simulink model "Test3"  (R2018b)
settings: Solver=VariableStepAuto  StartTime=0.0  StopTime=5e-6  RelTol=1e-3
model workspace (MAT data in the model file):
  a_1 = 0
  a_2 = 0
  delta = 0.001
values from neighbouring files (symbols this model uses):
  A = 1e-6    (= 1e-06)    [IC_4DOF_new.m]    (also in IC_4DOF_new2.m; ODE_4DOF_new.m = [zeros(4), eye(4); C+Hs, omega_dim*G+Hd/omega_dim]; ODE_MAGLEV_4DOF.m = [zeros(4), eye(4); C+Hs, (omega_dim*G)+(Hd/omega_dim)]; PID_Test2_.m = [zeros(4), eye(4); C+Hs, (omega_dim*G)+(Hd/omega_dim)])
  a1_dim = a1/Sl    (= 0.409090909091)    [IC_4DOF_new.m]    (also in IC_4DOF_new2.m; PID_Test2_.m; var_IC_4DOF.m)
  a2_dim = a2/Sl    (= 0.409090909091)    [IC_4DOF_new.m]    (also in IC_4DOF_new2.m; PID_Test2_.m; var_IC_4DOF.m)
  Ax_dim = Ax/Sf    (= 0.000833333333333)    [IC_4DOF_new.m]    (also in IC_4DOF_new2.m; PID_Test2_.m; var_IC_4DOF.m)
  delta_dim = delta_dim/Sx    (= 1)    [IC_4DOF_new.m]    (also in IC_4DOF_new2.m; PID_Test2_.m; var_IC_4DOF.m)
  h = 0.2*1e-3    (= 0.0002)    [IC_4DOF_new.m]    (also in IC_4DOF_new2.m; PID_Test2_.m; var_IC_4DOF.m)
  h_dim = h/Sl    (= 0.00909090909091)    [IC_4DOF_new.m]    (also in IC_4DOF_new2.m; PID_Test2_.m; var_IC_4DOF.m)
  i0_dim = i0/Si    (= 0)    [IC_4DOF_new.m]    (also in IC_4DOF_new2.m = 0.05; PID_Test2_.m = 0.0007; var_IC_4DOF.m = 0.5)
  omega_dim = omega/Sw    [IC_4DOF_new.m]    (also in IC_4DOF_new2.m; ODE_4DOF_new.m = par(11); ODE_MAGLEV_4DOF.m = par(11); PID_Test2_.m)
  P2 = par(22)    [Force_4DOF.m]    (also in IC_4DOF_new.m = 2.178; IC_4DOF_new2.m = 2.178; PID_Test2_.m = 8.714; var_IC_4DOF.m = 2.178)
  p_dim = nu*2*pi/Sw    [AFC_4DOF_NM.m]    (also in IC_4DOF_new.m = p/Sw; IC_4DOF_new2.m = p/Sw; PID_Test2_.m = p/Sw; var_IC_4DOF.m = p/Sw)
  Pk = par(15)    [Force_4DOF.m]    (also in IC_4DOF_new.m = 8.41666666667e-05; IC_4DOF_new2.m = ka*P_e/(cm*R_e*delta_dim^3); PID_Test2_.m = 1000000; var_IC_4DOF.m = ka*P_e/(cm*R_e*delta_dim^3))
  Px_dim = Px/Sf    (= 0)    [IC_4DOF_new.m]    (also in IC_4DOF_new2.m = 1.62337662338; PID_Test2_.m; var_IC_4DOF.m)
  Zb = [1 0 0 -a1_dim ... (first row only)    [IC_4DOF_new.m]    (also in IC_4DOF_new2.m; PID_Test2_.m; var_IC_4DOF.m)
libraries: simulink x25, cstblocks x1, neural x1
settings Model: Creator=Vladimir  LastModifiedBy=first
settings SolverCC: AlgebraicLoopSolver=LineSearch

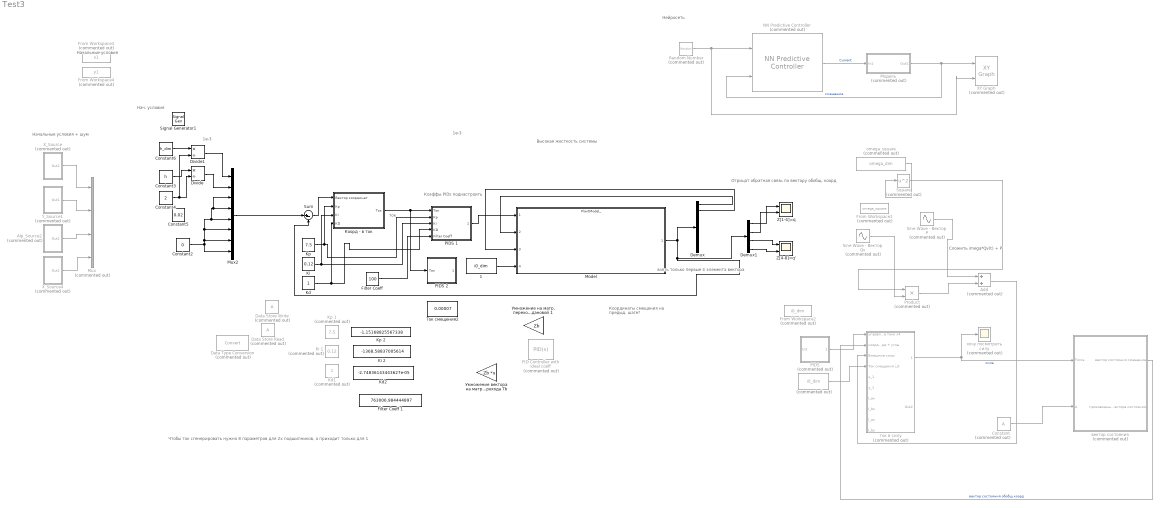
== system Test3 ==
  note: 1e-3
  note: Нач. условия
  note: 1e-3
  note: Высокая жесткость системы
  note: Коэффы PIDs поднастроить
  note: Чтобы ток сгенерировать нужно 8 параметров для 2х подшипников, а приходит только для 1
  note: Координаты смещения
      | на предыд. шаге?
  note: взять только первые 4 элемента вектора
  note: Нейросеть
  note: Начальные условия
  note: Отрицат обратная связь по вектору обобщ. коорд
  note: Сложить imega*Qv(t) + P
  note: Начальные условия + шум
  note: ток
  " " : Constant  Commented=on  Value=i0_dim
  " 1" : Constant  Value=i0_dim
  " Ток смещения2" : Constant  Value=0.00007
  " вектор состояния " : Subsystem  Commented=on
  Add : Sum  Commented=on
  Alp_Source2 : Subsystem  Commented=on
  Constant : Constant  Commented=on  Value=A
  Constant2 : Constant  Value=0
  Constant3 : Constant  Value=h
  Constant4 : Constant  Value=2
  Constant5 : Constant  Value=0.02
  Constant6 : Constant  Value=h_dim
  Data Store Read : DataStoreRead  Commented=on
  Data Store Write : DataStoreWrite  Commented=on
  Data Type Conversion : DataTypeConversion  Commented=on
  Demux : Demux  Outputs=8
  Demux1 : Demux
  Divide : Product  Inputs=*/
  Divide1 : Product  Inputs=*/
  "Filter Coeff " : Constant  Value=100
  Filter Coeff 1 : Constant  Value=763006.984444897
  From Workspace1 : FromWorkspace  Commented=on  VariableName=omega_square  SampleTime=0
  From Workspace2 : FromWorkspace  Commented=on  VariableName=i0_dim  SampleTime=0
  From Workspace3 : FromWorkspace  Commented=on  VariableName=x1  SampleTime=0
  From Workspace4 : FromWorkspace  Commented=on  VariableName=y1  SampleTime=0
  Kd : Constant
  Kd1 : Constant  Commented=on
  Kd2 : Constant  Value=-2.74836143443627e-05
  "Ki " : Constant  Value=0.12
  Ki 1 : Constant  Commented=on  Value=0.12
  Ki 2 : Constant  Value=-1368.58837005614
  "Kp " : Constant  Value=7.5
  Kp 1 : Constant  Commented=on  Value=7.5
  Kp 2 : Constant  Value=-1.15168825567338
  Model : ModelReference  ModelNameDialog=PlantModel_.slx  SimulationMode=Normal  ModelReferenceVersion=1.31
  Mux : Mux  Commented=on
  Mux2 : Mux  Inputs=8
  NN Predictive Controller : neural/Control Systems/NN Predictive Controller  Commented=on  epochs=500  minp=[]  maxp=[]  mint=[]  maxt=[]  Normalize=[]  IW=[]  LW1_2=[]  LW2_1=[]  B1=[]  B2=[]  max_i_int=[]  min_i_int=[]  limit_output=[]  max_output=[]  min_output=[]  Use_Previous_Weights=[]  N2=7  Nu=2  Ts=[]  rho=0.05  alpha=0.001  csrchfun=csrchbac  maxiter=2  S1=[]  Ni=[]  Nj=[]  sim_file=0  trainfun=trainlm  Use_validation=[]  Use_Testing=[]  max_i=[]  min_i=[]  sam_training=[]
      settings: SourceProductName=Neural Network Toolbox  SourceProductBaseCode=NN
  "PID Controller with ideal coeff " : simulink/Continuous/PID Controller  Commented=on  Controller=PID  Form=Parallel  TimeDomain=Continuous-time  SampleTime=-1  IntegratorMethod=Forward Euler  FilterMethod=Forward Euler  ControllerParametersSource=internal  P=7.5  I=0.12  D=1  UseFilter=on  N=100  TunerSelectOption=Transfer Function Based (PID Tuner App)  InitialConditionSource=internal  InitialConditionForIntegrator=0  InitialConditionForFilter=0  DifferentiatorICPrevScaledInput=0  ExternalReset=none  TrackingMode=off  Kt=1  LimitOutput=off  UpperSaturationLimit=inf  LowerSaturationLimit=-inf  LinearizeAsGain=on  AntiWindupMode=none  Kb=1  POutMin=[]  POutMax=[]  IOutMin=[]  IOutMax=[]  DOutMin=[]  DOutMax=[]  NOutMin=[]  NOutMax=[]  SumOutMin=[]  SumOutMax=[]  SaturationOutMin=[]  SaturationOutMax=[]  PParamMin=[]  PParamMax=[]  IParamMin=[]  IParamMax=[]  DParamMin=[]  DParamMax=[]  NParamMin=[]  NParamMax=[]  KbParamMin=[]  KbParamMax=[]  KtParamMin=[]  KtParamMax=[]  KbOutMin=[]  KbOutMax=[]  KtOutMin=[]  KtOutMax=[]  IntegratorOutMin=[]  IntegratorOutMax=[]  FilterOutMin=[]  FilterOutMax=[]  SumI1OutMin=[]  SumI1OutMax=[]  SumI2OutMin=[]  SumI2OutMax=[]  SumI3OutMin=[]  SumI3OutMax=[]  SumI4OutMin=[]  SumI4OutMax=[]  SumDOutMin=[]  SumDOutMax=[]  DifferentiatorOutMin=[]  DifferentiatorOutMax=[]  FilterDiffOutCoefMin=[]  FilterDiffOutCoefMax=[]  ReciprocalOutMin=[]  ReciprocalOutMax=[]  SumDenOutMin=[]  SumDenOutMax=[]  SumNumOutMin=[]  SumNumOutMax=[]  DivideOutMin=[]  DivideOutMax=[]  IntegratorContinuousStateAttributes=''  IntegratorStateMustResolveToSignalObject=off  IntegratorRTWStateStorageClass=Auto  FilterContinuousStateAttributes=''  FilterStateMustResolveToSignalObject=off  FilterRTWStateStorageClass=Auto  ParallelPVariant=InternalParameters  IdealPVariant=Disabled  IVariant=InternalParameters  DVariant=InternalParameters  IntegratorVariant=Continuous  SatVariant=Disabled  AWVariant=Passthrough  PCopyVariant=Disabled  TRVariant=Disabled  FdbkBlocksVariant=Forward  IdealPFdbkVariant=Disabled  SatFdbkVariant=Disabled  DerivativeFilterVariant=ContFilter  NVariant=InternalParameters  NCopyVariant=Disabled  FilterICVariant=InternalICsFilter  IntegratorICVariant=InternalICs  ExternalResetVariant=Disabled  TRSumVariant=Passthrough  SumFdbkVariant=Disabled  SumVariant=Sum_PID
  "PIDS " : Subsystem  Commented=on
  PIDS 1 : Subsystem
  PIDS 2 : Subsystem
  Product : Product  Commented=on
  Random Number : RandomNumber  Commented=on  SampleTime=0.1
  Signal Generator1 : SignalGenerator  Amplitude=h/2  Units=rad/sec
  Sine Wave - Вектор P : Sin  Commented=on  Amplitude=Ax_dim  Bias=Px_dim  Frequency=p_dim  SampleTime=1
  Sine Wave - Вектор Qv : Sin  Commented=on  Amplitude=Ax_dim  Bias=Px_dim  Frequency=p_dim  SampleTime=1
  Square : Math  Commented=on  Operator=square  SaturateOnIntegerOverflow=on
  Sum : Sum  Inputs=|+-
  XY Graph : simulink/Sinks/XY Graph  Commented=on  xmin=-1  xmax=1  ymin=-1  ymax=1  st=-1
  X_Source : Subsystem  Commented=on
  X_Source4 : Subsystem  Commented=on
  Y_Source1 : Subsystem  Commented=on
  "Z[1-4]=q " : Scope  NumInputPorts=2
  Z[4-8]=q' : Scope  NumInputPorts=2
  omega_square : Constant  Commented=on  Value=omega_dim
  "Коорд - в ток " : Subsystem
  "Модель " : Subsystem  Commented=on
  "Умножение вектора на матр. перехода Tb " : Gain  Gain=Zb  Multiplication=Matrix(K*u) (u vector)
  "Умножение на матр. перехода Tb, посмотреть у Богдановой 1" : Gain  Gain=Zb
  "ток в силу " : Subsystem  Commented=on
  хочу посмотреть силу : Scope  Commented=on
  wires:
  X_Source/1(Out1) -> Mux/1
  Y_Source1/1(Out1) -> Mux/2
  Alp_Source2/1(Out1) -> Mux/3
  X_Source4/1(Out1) -> Mux/4
  " вектор состояния "/1(вектор состояния смещение) -> "ток в силу "/2(координаты на предидущий такт коорд + углы)  "вектор состояния обобщ коорд"
  "ток в силу "/1(" ") -> хочу посмотреть силу/1, " вектор состояния "/1(Force)  "сила"
  Demux1/1 -> "Z[1-4]=q "/1
  Demux1/2 -> "Z[1-4]=q "/2
  Demux1/3 -> Z[4-8]=q'/1
  Demux1/4 -> Z[4-8]=q'/2
  Add/1 -> "ток в силу "/3(Внешние силы)
  Sine Wave - Вектор P/1 -> Add/1
  "PIDS "/1("  ") -> "ток в силу "/1(управляющие токи x4)
  Sine Wave - Вектор Qv/1 -> Product/2
  Product/1 -> Add/2
  " "/1 -> "ток в силу "/4(Ток смещения i_0)
  Constant/1 -> " вектор состояния "/2("A ")
  omega_square/1 -> Square/1
  Square/1 -> Product/1
  Sum/1 -> "Коорд - в ток "/1(Вектор координат)
  Random Number/1 -> XY Graph/2, NN Predictive Controller/1
  NN Predictive Controller/1 -> "Модель "/1(In1)  "Current"
  "Модель "/1(Out1) -> NN Predictive Controller/2, XY Graph/1  "смещение"
  Model/1 -> Demux1/1, Sum/2, Demux/1
  "Коорд - в ток "/1(Ток) -> PIDS 2/1(Ток), PIDS 1/1(Ток)
  Demux/1 -> Model/2
  Demux/2 -> Model/3
  Constant2/1 -> Mux2/8, Mux2/6, Mux2/3, Mux2/4, Mux2/5, Mux2/7
  Mux2/1 -> Sum/1
  Constant4/1 -> Divide1/2, Divide/2
  "Kp "/1 -> "Коорд - в ток "/2(Kp), PIDS 1/2(Kp)
  "Ki "/1 -> PIDS 1/3(Ki), "Коорд - в ток "/3(Ki)
  Kd/1 -> PIDS 1/4("KD "), "Коорд - в ток "/4("KD ")
  "Filter Coeff "/1 -> PIDS 1/5(Filter Coeff)
  " 1"/1 -> Model/4
  PIDS 1/1("  ") -> Model/1
  Constant3/1 -> Divide/1
  Constant6/1 -> Divide1/1
  Divide1/1 -> Mux2/1
  Divide/1 -> Mux2/2

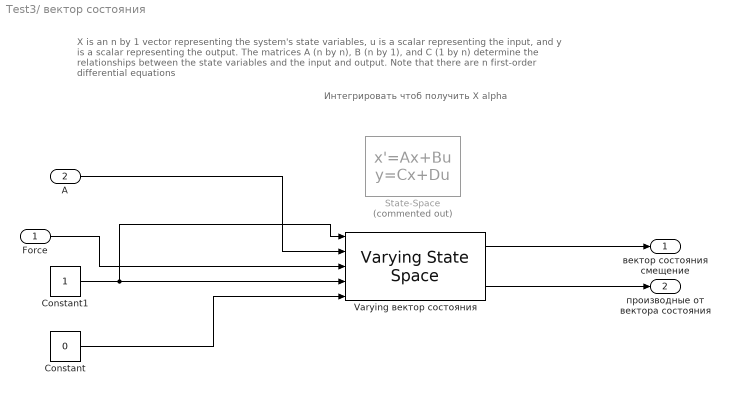
== system Test3/ вектор состояния  ==
  note: X is an n by 1 vector representing the system's state variables, u is a scalar representing the input, and y is a scalar representing the output.
      |  The matrices A (n by n), B (n by 1), and C (1 by n) determine the relationships between the state variables and the input and output.
      | Note that there are n first-order differential equations
  note: Интегрировать чтоб получить X alpha
  Force : Inport
  "A " : Inport  Port=2
  Constant : Constant  Value=0
  Constant1 : Constant
  State-Space : StateSpace  Commented=on  InitialCondition=0
  Varying вектор состояния : cstblocks/Linear Parameter Varying/Varying State Space  x0=0  xNames=''  OutputX=on  OutputDX=on
      settings: SourceProductName=Control System Toolbox
  вектор состояния смещение : Outport
  производные от вектора состояния : Outport  Port=2
  wires:
  Force/1 -> Varying вектор состояния/3
  "A "/1 -> Varying вектор состояния/2
  Varying вектор состояния/3 -> производные от вектора состояния/1
  Constant/1 -> Varying вектор состояния/5
  Constant1/1 -> Varying вектор состояния/4, Varying вектор состояния/1
  Varying вектор состояния/1 -> вектор состояния смещение/1

== system Test3/Alp_Source2 ==
  note: Tok Here
  note: dtrnjh 4[
  Band-Limited White Noise : simulink/Sources/Band-Limited White Noise  Cov=[0.1]  Ts=0.1  seed=[23341]
  Gain : Gain
  Gain1 : Gain
  Sine Wave : Sin  SampleTime=0
  Step : Step  SampleTime=0
  Sum : Sum  Inputs=|+++
  Out1 : Outport
  wires:
  Gain1/1 -> Sum/3
  Band-Limited White Noise/1 -> Gain/1
  Sine Wave/1 -> Gain1/1
  Step/1 -> Sum/1
  Gain/1 -> Sum/2
  Sum/1 -> Out1/1

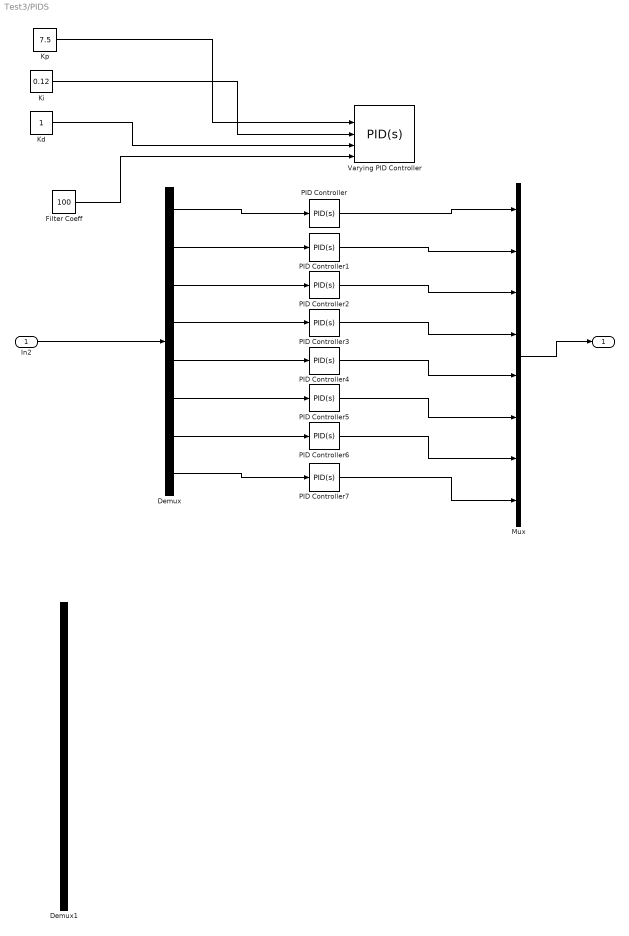
== system Test3/PIDS  ==
  In2 : Inport
  Demux : Demux  Outputs=8
  Demux1 : Demux  Outputs=8
  "Filter Coeff " : Constant  Value=100
  Kd : Constant
  "Ki " : Constant  Value=0.12
  "Kp " : Constant  Value=7.5
  Mux : Mux  Inputs=8
  PID Controller{,1..7} (8 alike) : simulink/Continuous/PID Controller  Controller=PID  Form=Parallel  TimeDomain=Continuous-time  SampleTime=-1  IntegratorMethod=Forward Euler  FilterMethod=Forward Euler  ControllerParametersSource=internal  P=1  I=1  D=0  UseFilter=on  N=100  TunerSelectOption=Transfer Function Based (PID Tuner App)  InitialConditionSource=internal  InitialConditionForIntegrator=0  InitialConditionForFilter=0  DifferentiatorICPrevScaledInput=0  ExternalReset=none  TrackingMode=off  Kt=1  LimitOutput=off  UpperSaturationLimit=inf  LowerSaturationLimit=-inf  LinearizeAsGain=on  AntiWindupMode=none  Kb=1  POutMin=[]  POutMax=[]  IOutMin=[]  IOutMax=[]  DOutMin=[]  DOutMax=[]  NOutMin=[]  NOutMax=[]  SumOutMin=[]  SumOutMax=[]  SaturationOutMin=[]  SaturationOutMax=[]  PParamMin=[]  PParamMax=[]  IParamMin=[]  IParamMax=[]  DParamMin=[]  DParamMax=[]  NParamMin=[]  NParamMax=[]  KbParamMin=[]  KbParamMax=[]  KtParamMin=[]  KtParamMax=[]  KbOutMin=[]  KbOutMax=[]  KtOutMin=[]  KtOutMax=[]  IntegratorOutMin=[]  IntegratorOutMax=[]  FilterOutMin=[]  FilterOutMax=[]  SumI1OutMin=[]  SumI1OutMax=[]  SumI2OutMin=[]  SumI2OutMax=[]  SumI3OutMin=[]  SumI3OutMax=[]  SumI4OutMin=[]  SumI4OutMax=[]  SumDOutMin=[]  SumDOutMax=[]  DifferentiatorOutMin=[]  DifferentiatorOutMax=[]  FilterDiffOutCoefMin=[]  FilterDiffOutCoefMax=[]  ReciprocalOutMin=[]  ReciprocalOutMax=[]  SumDenOutMin=[]  SumDenOutMax=[]  SumNumOutMin=[]  SumNumOutMax=[]  DivideOutMin=[]  DivideOutMax=[]  IntegratorContinuousStateAttributes=''  IntegratorStateMustResolveToSignalObject=off  IntegratorRTWStateStorageClass=Auto  FilterContinuousStateAttributes=''  FilterStateMustResolveToSignalObject=off  FilterRTWStateStorageClass=Auto  ParallelPVariant=InternalParameters  IdealPVariant=Disabled  IVariant=InternalParameters  DVariant=InternalParameters  IntegratorVariant=Continuous  SatVariant=Disabled  AWVariant=Passthrough  PCopyVariant=Disabled  TRVariant=Disabled  FdbkBlocksVariant=Forward  IdealPFdbkVariant=Disabled  SatFdbkVariant=Disabled  DerivativeFilterVariant=ContFilter  NVariant=InternalParameters  NCopyVariant=Disabled  FilterICVariant=InternalICsFilter  IntegratorICVariant=InternalICs  ExternalResetVariant=Disabled  TRSumVariant=Passthrough  SumFdbkVariant=Disabled  SumVariant=Sum_PID
  Varying PID Controller : simulink/Continuous/PID Controller  Controller=PID  Form=Parallel  TimeDomain=Continuous-time  SampleTime=-1  IntegratorMethod=Forward Euler  FilterMethod=Forward Euler  ControllerParametersSource=external  P=1  I=1  D=0  UseFilter=on  N=100  TunerSelectOption=Transfer Function Based (PID Tuner App)  InitialConditionSource=internal  InitialConditionForIntegrator=0  InitialConditionForFilter=0  DifferentiatorICPrevScaledInput=0  ExternalReset=none  TrackingMode=off  Kt=1  LimitOutput=off  UpperSaturationLimit=inf  LowerSaturationLimit=-inf  LinearizeAsGain=on  AntiWindupMode=none  Kb=1  POutMin=[]  POutMax=[]  IOutMin=[]  IOutMax=[]  DOutMin=[]  DOutMax=[]  NOutMin=[]  NOutMax=[]  SumOutMin=[]  SumOutMax=[]  SaturationOutMin=[]  SaturationOutMax=[]  PParamMin=[]  PParamMax=[]  IParamMin=[]  IParamMax=[]  DParamMin=[]  DParamMax=[]  NParamMin=[]  NParamMax=[]  KbParamMin=[]  KbParamMax=[]  KtParamMin=[]  KtParamMax=[]  KbOutMin=[]  KbOutMax=[]  KtOutMin=[]  KtOutMax=[]  IntegratorOutMin=[]  IntegratorOutMax=[]  FilterOutMin=[]  FilterOutMax=[]  SumI1OutMin=[]  SumI1OutMax=[]  SumI2OutMin=[]  SumI2OutMax=[]  SumI3OutMin=[]  SumI3OutMax=[]  SumI4OutMin=[]  SumI4OutMax=[]  SumDOutMin=[]  SumDOutMax=[]  DifferentiatorOutMin=[]  DifferentiatorOutMax=[]  FilterDiffOutCoefMin=[]  FilterDiffOutCoefMax=[]  ReciprocalOutMin=[]  ReciprocalOutMax=[]  SumDenOutMin=[]  SumDenOutMax=[]  SumNumOutMin=[]  SumNumOutMax=[]  DivideOutMin=[]  DivideOutMax=[]  IntegratorContinuousStateAttributes=''  IntegratorStateMustResolveToSignalObject=off  IntegratorRTWStateStorageClass=Auto  FilterContinuousStateAttributes=''  FilterStateMustResolveToSignalObject=off  FilterRTWStateStorageClass=Auto  ParallelPVariant=ExternalParameters  IdealPVariant=Disabled  IVariant=ExternalParameters  DVariant=ExternalParameters  IntegratorVariant=Continuous  SatVariant=Disabled  AWVariant=Passthrough  PCopyVariant=Disabled  TRVariant=Disabled  FdbkBlocksVariant=Forward  IdealPFdbkVariant=Disabled  SatFdbkVariant=Disabled  DerivativeFilterVariant=ContFilter  NVariant=ExternalParameters  NCopyVariant=Disabled  FilterICVariant=InternalICsFilter  IntegratorICVariant=InternalICs  ExternalResetVariant=Disabled  TRSumVariant=Passthrough  SumFdbkVariant=Disabled  SumVariant=Sum_PID
  "  " : Outport
  wires:
  Demux/1 -> PID Controller/1
  Demux/2 -> PID Controller1/1
  Demux/3 -> PID Controller2/1
  Demux/4 -> PID Controller3/1
  In2/1 -> Demux/1
  Demux/5 -> PID Controller4/1
  Demux/6 -> PID Controller5/1
  Demux/7 -> PID Controller6/1
  Demux/8 -> PID Controller7/1
  PID Controller/1 -> Mux/1
  PID Controller1/1 -> Mux/2
  PID Controller2/1 -> Mux/3
  PID Controller3/1 -> Mux/4
  PID Controller4/1 -> Mux/5
  PID Controller5/1 -> Mux/6
  PID Controller6/1 -> Mux/7
  PID Controller7/1 -> Mux/8
  Mux/1 -> "  "/1
  "Kp "/1 -> Varying PID Controller/2
  "Filter Coeff "/1 -> Varying PID Controller/5
  "Ki "/1 -> Varying PID Controller/3
  Kd/1 -> Varying PID Controller/4

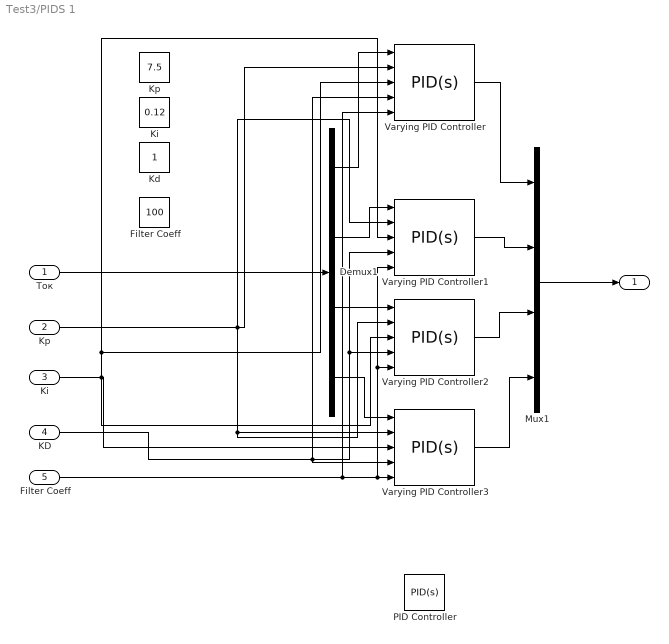
== system Test3/PIDS 1 ==
  Ток : Inport
  Kp : Inport  Port=2
  Ki : Inport  Port=3
  "KD " : Inport  Port=4
  Filter Coeff : Inport  Port=5
  Demux1 : Demux
  "Filter Coeff " : Constant  Value=100
  Kd : Constant
  "Ki " : Constant  Value=0.12
  "Kp " : Constant  Value=7.5
  Mux1 : Mux
  PID Controller : simulink/Continuous/PID Controller  Controller=PID  Form=Parallel  TimeDomain=Continuous-time  SampleTime=-1  IntegratorMethod=Forward Euler  FilterMethod=Forward Euler  ControllerParametersSource=internal  P=1  I=1  D=0  UseFilter=on  N=100  TunerSelectOption=Transfer Function Based (PID Tuner App)  InitialConditionSource=internal  InitialConditionForIntegrator=0  InitialConditionForFilter=0  DifferentiatorICPrevScaledInput=0  ExternalReset=none  TrackingMode=off  Kt=1  LimitOutput=off  UpperSaturationLimit=inf  LowerSaturationLimit=-inf  LinearizeAsGain=on  AntiWindupMode=none  Kb=1  POutMin=[]  POutMax=[]  IOutMin=[]  IOutMax=[]  DOutMin=[]  DOutMax=[]  NOutMin=[]  NOutMax=[]  SumOutMin=[]  SumOutMax=[]  SaturationOutMin=[]  SaturationOutMax=[]  PParamMin=[]  PParamMax=[]  IParamMin=[]  IParamMax=[]  DParamMin=[]  DParamMax=[]  NParamMin=[]  NParamMax=[]  KbParamMin=[]  KbParamMax=[]  KtParamMin=[]  KtParamMax=[]  KbOutMin=[]  KbOutMax=[]  KtOutMin=[]  KtOutMax=[]  IntegratorOutMin=[]  IntegratorOutMax=[]  FilterOutMin=[]  FilterOutMax=[]  SumI1OutMin=[]  SumI1OutMax=[]  SumI2OutMin=[]  SumI2OutMax=[]  SumI3OutMin=[]  SumI3OutMax=[]  SumI4OutMin=[]  SumI4OutMax=[]  SumDOutMin=[]  SumDOutMax=[]  DifferentiatorOutMin=[]  DifferentiatorOutMax=[]  FilterDiffOutCoefMin=[]  FilterDiffOutCoefMax=[]  ReciprocalOutMin=[]  ReciprocalOutMax=[]  SumDenOutMin=[]  SumDenOutMax=[]  SumNumOutMin=[]  SumNumOutMax=[]  DivideOutMin=[]  DivideOutMax=[]  IntegratorContinuousStateAttributes=''  IntegratorStateMustResolveToSignalObject=off  IntegratorRTWStateStorageClass=Auto  FilterContinuousStateAttributes=''  FilterStateMustResolveToSignalObject=off  FilterRTWStateStorageClass=Auto  ParallelPVariant=InternalParameters  IdealPVariant=Disabled  IVariant=InternalParameters  DVariant=InternalParameters  IntegratorVariant=Continuous  SatVariant=Disabled  AWVariant=Passthrough  PCopyVariant=Disabled  TRVariant=Disabled  FdbkBlocksVariant=Forward  IdealPFdbkVariant=Disabled  SatFdbkVariant=Disabled  DerivativeFilterVariant=ContFilter  NVariant=InternalParameters  NCopyVariant=Disabled  FilterICVariant=InternalICsFilter  IntegratorICVariant=InternalICs  ExternalResetVariant=Disabled  TRSumVariant=Passthrough  SumFdbkVariant=Disabled  SumVariant=Sum_PID
  Varying PID Controller{,1..3} (4 alike) : simulink/Continuous/PID Controller  Controller=PID  Form=Parallel  TimeDomain=Continuous-time  SampleTime=-1  IntegratorMethod=Forward Euler  FilterMethod=Forward Euler  ControllerParametersSource=external  P=1  I=1  D=0  UseFilter=on  N=100  TunerSelectOption=Transfer Function Based (PID Tuner App)  InitialConditionSource=internal  InitialConditionForIntegrator=0  InitialConditionForFilter=0  DifferentiatorICPrevScaledInput=0  ExternalReset=none  TrackingMode=off  Kt=1  LimitOutput=off  UpperSaturationLimit=inf  LowerSaturationLimit=-inf  LinearizeAsGain=on  AntiWindupMode=none  Kb=1  POutMin=[]  POutMax=[]  IOutMin=[]  IOutMax=[]  DOutMin=[]  DOutMax=[]  NOutMin=[]  NOutMax=[]  SumOutMin=[]  SumOutMax=[]  SaturationOutMin=[]  SaturationOutMax=[]  PParamMin=[]  PParamMax=[]  IParamMin=[]  IParamMax=[]  DParamMin=[]  DParamMax=[]  NParamMin=[]  NParamMax=[]  KbParamMin=[]  KbParamMax=[]  KtParamMin=[]  KtParamMax=[]  KbOutMin=[]  KbOutMax=[]  KtOutMin=[]  KtOutMax=[]  IntegratorOutMin=[]  IntegratorOutMax=[]  FilterOutMin=[]  FilterOutMax=[]  SumI1OutMin=[]  SumI1OutMax=[]  SumI2OutMin=[]  SumI2OutMax=[]  SumI3OutMin=[]  SumI3OutMax=[]  SumI4OutMin=[]  SumI4OutMax=[]  SumDOutMin=[]  SumDOutMax=[]  DifferentiatorOutMin=[]  DifferentiatorOutMax=[]  FilterDiffOutCoefMin=[]  FilterDiffOutCoefMax=[]  ReciprocalOutMin=[]  ReciprocalOutMax=[]  SumDenOutMin=[]  SumDenOutMax=[]  SumNumOutMin=[]  SumNumOutMax=[]  DivideOutMin=[]  DivideOutMax=[]  IntegratorContinuousStateAttributes=''  IntegratorStateMustResolveToSignalObject=off  IntegratorRTWStateStorageClass=Auto  FilterContinuousStateAttributes=''  FilterStateMustResolveToSignalObject=off  FilterRTWStateStorageClass=Auto  ParallelPVariant=ExternalParameters  IdealPVariant=Disabled  IVariant=ExternalParameters  DVariant=ExternalParameters  IntegratorVariant=Continuous  SatVariant=Disabled  AWVariant=Passthrough  PCopyVariant=Disabled  TRVariant=Disabled  FdbkBlocksVariant=Forward  IdealPFdbkVariant=Disabled  SatFdbkVariant=Disabled  DerivativeFilterVariant=ContFilter  NVariant=ExternalParameters  NCopyVariant=Disabled  FilterICVariant=InternalICsFilter  IntegratorICVariant=InternalICs  ExternalResetVariant=Disabled  TRSumVariant=Passthrough  SumFdbkVariant=Disabled  SumVariant=Sum_PID
  "  " : Outport
  wires:
  Mux1/1 -> "  "/1
  Ток/1 -> Demux1/1
  Demux1/1 -> Varying PID Controller/1
  Varying PID Controller/1 -> Mux1/1
  Demux1/2 -> Varying PID Controller1/1
  Varying PID Controller1/1 -> Mux1/2
  Demux1/3 -> Varying PID Controller2/1
  Varying PID Controller2/1 -> Mux1/3
  Demux1/4 -> Varying PID Controller3/1
  Varying PID Controller3/1 -> Mux1/4
  Filter Coeff/1 -> Varying PID Controller/5, Varying PID Controller1/5, Varying PID Controller2/5, Varying PID Controller3/5
  "KD "/1 -> Varying PID Controller/4, Varying PID Controller1/4, Varying PID Controller2/4, Varying PID Controller3/4
  Ki/1 -> Varying PID Controller/3, Varying PID Controller1/3, Varying PID Controller2/3, Varying PID Controller3/3
  Kp/1 -> Varying PID Controller3/2, Varying PID Controller2/2, Varying PID Controller1/2, Varying PID Controller/2

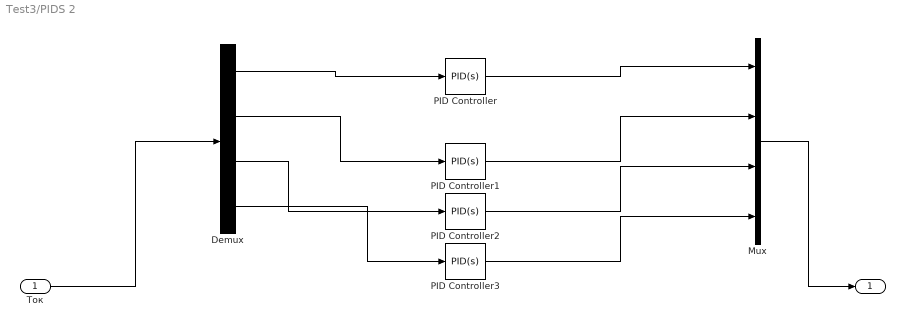
== system Test3/PIDS 2 ==
  Ток : Inport
  Demux : Demux
  Mux : Mux
  PID Controller : simulink/Continuous/PID Controller  Controller=PID  Form=Parallel  TimeDomain=Continuous-time  SampleTime=-1  IntegratorMethod=Forward Euler  FilterMethod=Forward Euler  ControllerParametersSource=internal  P=-1.15168825567338  I=-1368.58837005614  D=-2.74836143443627e-05  UseFilter=on  N=763006.984444897  TunerSelectOption=Transfer Function Based (PID Tuner App)  InitialConditionSource=internal  InitialConditionForIntegrator=0  InitialConditionForFilter=0  DifferentiatorICPrevScaledInput=0  ExternalReset=none  TrackingMode=off  Kt=1  LimitOutput=off  UpperSaturationLimit=inf  LowerSaturationLimit=-inf  LinearizeAsGain=on  AntiWindupMode=none  Kb=1  POutMin=[]  POutMax=[]  IOutMin=[]  IOutMax=[]  DOutMin=[]  DOutMax=[]  NOutMin=[]  NOutMax=[]  SumOutMin=[]  SumOutMax=[]  SaturationOutMin=[]  SaturationOutMax=[]  PParamMin=[]  PParamMax=[]  IParamMin=[]  IParamMax=[]  DParamMin=[]  DParamMax=[]  NParamMin=[]  NParamMax=[]  KbParamMin=[]  KbParamMax=[]  KtParamMin=[]  KtParamMax=[]  KbOutMin=[]  KbOutMax=[]  KtOutMin=[]  KtOutMax=[]  IntegratorOutMin=[]  IntegratorOutMax=[]  FilterOutMin=[]  FilterOutMax=[]  SumI1OutMin=[]  SumI1OutMax=[]  SumI2OutMin=[]  SumI2OutMax=[]  SumI3OutMin=[]  SumI3OutMax=[]  SumI4OutMin=[]  SumI4OutMax=[]  SumDOutMin=[]  SumDOutMax=[]  DifferentiatorOutMin=[]  DifferentiatorOutMax=[]  FilterDiffOutCoefMin=[]  FilterDiffOutCoefMax=[]  ReciprocalOutMin=[]  ReciprocalOutMax=[]  SumDenOutMin=[]  SumDenOutMax=[]  SumNumOutMin=[]  SumNumOutMax=[]  DivideOutMin=[]  DivideOutMax=[]  IntegratorContinuousStateAttributes=''  IntegratorStateMustResolveToSignalObject=off  IntegratorRTWStateStorageClass=Auto  FilterContinuousStateAttributes=''  FilterStateMustResolveToSignalObject=off  FilterRTWStateStorageClass=Auto  ParallelPVariant=InternalParameters  IdealPVariant=Disabled  IVariant=InternalParameters  DVariant=InternalParameters  IntegratorVariant=Continuous  SatVariant=Disabled  AWVariant=Passthrough  PCopyVariant=Disabled  TRVariant=Disabled  FdbkBlocksVariant=Forward  IdealPFdbkVariant=Disabled  SatFdbkVariant=Disabled  DerivativeFilterVariant=ContFilter  NVariant=InternalParameters  NCopyVariant=Disabled  FilterICVariant=InternalICsFilter  IntegratorICVariant=InternalICs  ExternalResetVariant=Disabled  TRSumVariant=Passthrough  SumFdbkVariant=Disabled  SumVariant=Sum_PID
  PID Controller1 : simulink/Continuous/PID Controller  Controller=PID  Form=Parallel  TimeDomain=Continuous-time  SampleTime=-1  IntegratorMethod=Forward Euler  FilterMethod=Forward Euler  ControllerParametersSource=internal  P=-54.4337936545149  I=-10142312.4199932  D=1.54659232458287e-05  UseFilter=on  N=3519595.48675481  TunerSelectOption=Transfer Function Based (PID Tuner App)  InitialConditionSource=internal  InitialConditionForIntegrator=0  InitialConditionForFilter=0  DifferentiatorICPrevScaledInput=0  ExternalReset=none  TrackingMode=off  Kt=1  LimitOutput=off  UpperSaturationLimit=inf  LowerSaturationLimit=-inf  LinearizeAsGain=on  AntiWindupMode=none  Kb=1  POutMin=[]  POutMax=[]  IOutMin=[]  IOutMax=[]  DOutMin=[]  DOutMax=[]  NOutMin=[]  NOutMax=[]  SumOutMin=[]  SumOutMax=[]  SaturationOutMin=[]  SaturationOutMax=[]  PParamMin=[]  PParamMax=[]  IParamMin=[]  IParamMax=[]  DParamMin=[]  DParamMax=[]  NParamMin=[]  NParamMax=[]  KbParamMin=[]  KbParamMax=[]  KtParamMin=[]  KtParamMax=[]  KbOutMin=[]  KbOutMax=[]  KtOutMin=[]  KtOutMax=[]  IntegratorOutMin=[]  IntegratorOutMax=[]  FilterOutMin=[]  FilterOutMax=[]  SumI1OutMin=[]  SumI1OutMax=[]  SumI2OutMin=[]  SumI2OutMax=[]  SumI3OutMin=[]  SumI3OutMax=[]  SumI4OutMin=[]  SumI4OutMax=[]  SumDOutMin=[]  SumDOutMax=[]  DifferentiatorOutMin=[]  DifferentiatorOutMax=[]  FilterDiffOutCoefMin=[]  FilterDiffOutCoefMax=[]  ReciprocalOutMin=[]  ReciprocalOutMax=[]  SumDenOutMin=[]  SumDenOutMax=[]  SumNumOutMin=[]  SumNumOutMax=[]  DivideOutMin=[]  DivideOutMax=[]  IntegratorContinuousStateAttributes=''  IntegratorStateMustResolveToSignalObject=off  IntegratorRTWStateStorageClass=Auto  FilterContinuousStateAttributes=''  FilterStateMustResolveToSignalObject=off  FilterRTWStateStorageClass=Auto  ParallelPVariant=InternalParameters  IdealPVariant=Disabled  IVariant=InternalParameters  DVariant=InternalParameters  IntegratorVariant=Continuous  SatVariant=Disabled  AWVariant=Passthrough  PCopyVariant=Disabled  TRVariant=Disabled  FdbkBlocksVariant=Forward  IdealPFdbkVariant=Disabled  SatFdbkVariant=Disabled  DerivativeFilterVariant=ContFilter  NVariant=InternalParameters  NCopyVariant=Disabled  FilterICVariant=InternalICsFilter  IntegratorICVariant=InternalICs  ExternalResetVariant=Disabled  TRSumVariant=Passthrough  SumFdbkVariant=Disabled  SumVariant=Sum_PID
  PID Controller2 : simulink/Continuous/PID Controller  Controller=PID  Form=Parallel  TimeDomain=Continuous-time  SampleTime=-1  IntegratorMethod=Forward Euler  FilterMethod=Forward Euler  ControllerParametersSource=internal  P=1  I=1  D=0  UseFilter=on  N=100  TunerSelectOption=Transfer Function Based (PID Tuner App)  InitialConditionSource=internal  InitialConditionForIntegrator=0  InitialConditionForFilter=0  DifferentiatorICPrevScaledInput=0  ExternalReset=none  TrackingMode=off  Kt=1  LimitOutput=off  UpperSaturationLimit=inf  LowerSaturationLimit=-inf  LinearizeAsGain=on  AntiWindupMode=none  Kb=1  POutMin=[]  POutMax=[]  IOutMin=[]  IOutMax=[]  DOutMin=[]  DOutMax=[]  NOutMin=[]  NOutMax=[]  SumOutMin=[]  SumOutMax=[]  SaturationOutMin=[]  SaturationOutMax=[]  PParamMin=[]  PParamMax=[]  IParamMin=[]  IParamMax=[]  DParamMin=[]  DParamMax=[]  NParamMin=[]  NParamMax=[]  KbParamMin=[]  KbParamMax=[]  KtParamMin=[]  KtParamMax=[]  KbOutMin=[]  KbOutMax=[]  KtOutMin=[]  KtOutMax=[]  IntegratorOutMin=[]  IntegratorOutMax=[]  FilterOutMin=[]  FilterOutMax=[]  SumI1OutMin=[]  SumI1OutMax=[]  SumI2OutMin=[]  SumI2OutMax=[]  SumI3OutMin=[]  SumI3OutMax=[]  SumI4OutMin=[]  SumI4OutMax=[]  SumDOutMin=[]  SumDOutMax=[]  DifferentiatorOutMin=[]  DifferentiatorOutMax=[]  FilterDiffOutCoefMin=[]  FilterDiffOutCoefMax=[]  ReciprocalOutMin=[]  ReciprocalOutMax=[]  SumDenOutMin=[]  SumDenOutMax=[]  SumNumOutMin=[]  SumNumOutMax=[]  DivideOutMin=[]  DivideOutMax=[]  IntegratorContinuousStateAttributes=''  IntegratorStateMustResolveToSignalObject=off  IntegratorRTWStateStorageClass=Auto  FilterContinuousStateAttributes=''  FilterStateMustResolveToSignalObject=off  FilterRTWStateStorageClass=Auto  ParallelPVariant=InternalParameters  IdealPVariant=Disabled  IVariant=InternalParameters  DVariant=InternalParameters  IntegratorVariant=Continuous  SatVariant=Disabled  AWVariant=Passthrough  PCopyVariant=Disabled  TRVariant=Disabled  FdbkBlocksVariant=Forward  IdealPFdbkVariant=Disabled  SatFdbkVariant=Disabled  DerivativeFilterVariant=ContFilter  NVariant=InternalParameters  NCopyVariant=Disabled  FilterICVariant=InternalICsFilter  IntegratorICVariant=InternalICs  ExternalResetVariant=Disabled  TRSumVariant=Passthrough  SumFdbkVariant=Disabled  SumVariant=Sum_PID
  PID Controller3 : simulink/Continuous/PID Controller  Controller=PID  Form=Parallel  TimeDomain=Continuous-time  SampleTime=-1  IntegratorMethod=Forward Euler  FilterMethod=Forward Euler  ControllerParametersSource=internal  P=1  I=1  D=0  UseFilter=on  N=100  TunerSelectOption=Transfer Function Based (PID Tuner App)  InitialConditionSource=internal  InitialConditionForIntegrator=0  InitialConditionForFilter=0  DifferentiatorICPrevScaledInput=0  ExternalReset=none  TrackingMode=off  Kt=1  LimitOutput=off  UpperSaturationLimit=inf  LowerSaturationLimit=-inf  LinearizeAsGain=on  AntiWindupMode=none  Kb=1  POutMin=[]  POutMax=[]  IOutMin=[]  IOutMax=[]  DOutMin=[]  DOutMax=[]  NOutMin=[]  NOutMax=[]  SumOutMin=[]  SumOutMax=[]  SaturationOutMin=[]  SaturationOutMax=[]  PParamMin=[]  PParamMax=[]  IParamMin=[]  IParamMax=[]  DParamMin=[]  DParamMax=[]  NParamMin=[]  NParamMax=[]  KbParamMin=[]  KbParamMax=[]  KtParamMin=[]  KtParamMax=[]  KbOutMin=[]  KbOutMax=[]  KtOutMin=[]  KtOutMax=[]  IntegratorOutMin=[]  IntegratorOutMax=[]  FilterOutMin=[]  FilterOutMax=[]  SumI1OutMin=[]  SumI1OutMax=[]  SumI2OutMin=[]  SumI2OutMax=[]  SumI3OutMin=[]  SumI3OutMax=[]  SumI4OutMin=[]  SumI4OutMax=[]  SumDOutMin=[]  SumDOutMax=[]  DifferentiatorOutMin=[]  DifferentiatorOutMax=[]  FilterDiffOutCoefMin=[]  FilterDiffOutCoefMax=[]  ReciprocalOutMin=[]  ReciprocalOutMax=[]  SumDenOutMin=[]  SumDenOutMax=[]  SumNumOutMin=[]  SumNumOutMax=[]  DivideOutMin=[]  DivideOutMax=[]  IntegratorContinuousStateAttributes=''  IntegratorStateMustResolveToSignalObject=off  IntegratorRTWStateStorageClass=Auto  FilterContinuousStateAttributes=''  FilterStateMustResolveToSignalObject=off  FilterRTWStateStorageClass=Auto  ParallelPVariant=InternalParameters  IdealPVariant=Disabled  IVariant=InternalParameters  DVariant=InternalParameters  IntegratorVariant=Continuous  SatVariant=Disabled  AWVariant=Passthrough  PCopyVariant=Disabled  TRVariant=Disabled  FdbkBlocksVariant=Forward  IdealPFdbkVariant=Disabled  SatFdbkVariant=Disabled  DerivativeFilterVariant=ContFilter  NVariant=InternalParameters  NCopyVariant=Disabled  FilterICVariant=InternalICsFilter  IntegratorICVariant=InternalICs  ExternalResetVariant=Disabled  TRSumVariant=Passthrough  SumFdbkVariant=Disabled  SumVariant=Sum_PID
  "  " : Outport
  wires:
  Demux/2 -> PID Controller1/1
  Demux/3 -> PID Controller2/1
  Demux/4 -> PID Controller3/1
  Ток/1 -> Demux/1
  PID Controller1/1 -> Mux/2
  PID Controller2/1 -> Mux/3
  PID Controller3/1 -> Mux/4
  Mux/1 -> "  "/1
  PID Controller/1 -> Mux/1
  Demux/1 -> PID Controller/1

== system Test3/X_Source ==
  note: Tok Here
  note: dtrnjh 4[
  Band-Limited White Noise : simulink/Sources/Band-Limited White Noise  Cov=[0.1]  Ts=0.1  seed=[23341]
  Gain : Gain
  Gain1 : Gain
  Sine Wave : Sin  SampleTime=0
  Step : Step  SampleTime=0
  Sum : Sum  Inputs=|+++
  Out1 : Outport
  wires:
  Gain1/1 -> Sum/3
  Band-Limited White Noise/1 -> Gain/1
  Sine Wave/1 -> Gain1/1
  Step/1 -> Sum/1
  Gain/1 -> Sum/2
  Sum/1 -> Out1/1

== system Test3/X_Source4 ==
  note: Tok Here
  note: dtrnjh 4[
  Band-Limited White Noise : simulink/Sources/Band-Limited White Noise  Cov=[0.1]  Ts=0.1  seed=[23341]
  Gain : Gain
  Gain1 : Gain
  Sine Wave : Sin  SampleTime=0
  Step : Step  SampleTime=0
  Sum : Sum  Inputs=|+++
  Out1 : Outport
  wires:
  Gain1/1 -> Sum/3
  Band-Limited White Noise/1 -> Gain/1
  Sine Wave/1 -> Gain1/1
  Step/1 -> Sum/1
  Gain/1 -> Sum/2
  Sum/1 -> Out1/1

== system Test3/Y_Source1 ==
  note: Tok Here
  note: dtrnjh 4[
  Band-Limited White Noise : simulink/Sources/Band-Limited White Noise  Cov=[0.1]  Ts=0.1  seed=[23341]
  Gain : Gain
  Gain1 : Gain
  Ramp : simulink/Sources/Ramp  slope=1  start=0  InitialOutput=0
  Sine Wave : Sin  SampleTime=0
  Step : Step  SampleTime=0
  Sum : Sum  Inputs=|+++
  Out1 : Outport
  wires:
  Gain1/1 -> Sum/3
  Band-Limited White Noise/1 -> Gain/1
  Sine Wave/1 -> Gain1/1
  Step/1 -> Sum/1
  Gain/1 -> Sum/2
  Sum/1 -> Out1/1
  Ramp/1 -> ?

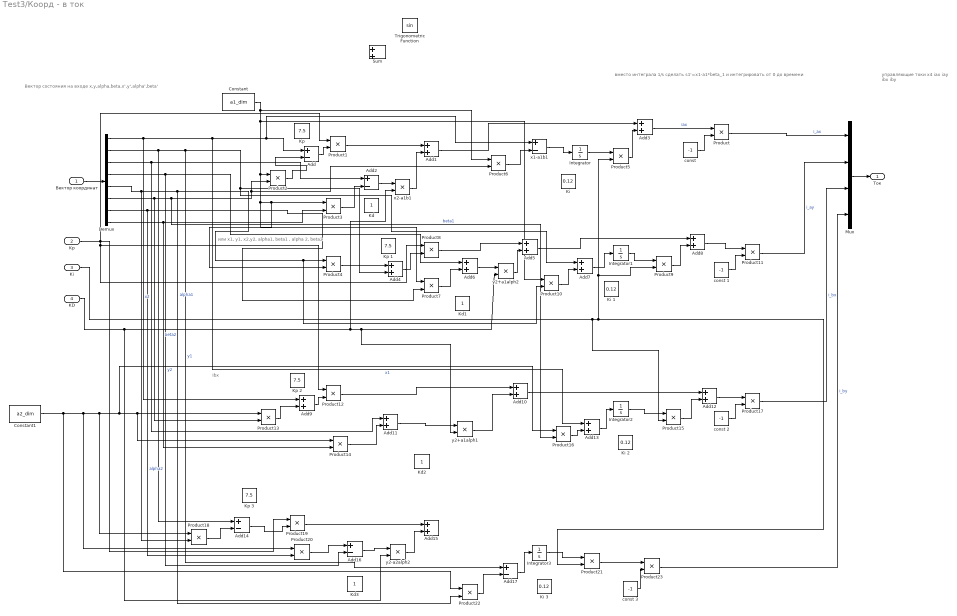
== system Test3/Коорд - в ток  ==
  note: вместо интеграла 1/s сделать s1'=x1-a1*beta_1 и интегрировать от 0 до времени
  note: Ibx
  note: или x1, y1, x2,y2, alpha1, beta1 , alpha 2, beta2
  note: управляющие токи x4
      | iax iay ibx iby
  note: Вектор состояния на входе x,y,alpha,beta,x',y',alpha',beta'
  Вектор координат : Inport
  Kp : Inport  Port=2
  Ki : Inport  Port=3
  "KD " : Inport  Port=4
  Add{,2,14,16..17} (5 alike) : Sum  Inputs=+-
  Add{1,3..13,15} (13 alike) : Sum
  Constant : Constant  Value=a1_dim
  Constant1 : Constant  Value=a2_dim
  Demux : Demux  Outputs=8
  Integrator : Integrator
  Integrator1 : Integrator
  Integrator2 : Integrator  UpperSaturationLimit=1  LowerSaturationLimit=0.001
  Integrator3 : Integrator
  Kd{,1..3} (4 alike) : Constant
  Ki {,1..3} (4 alike) : Constant  Value=0.12
  Kp {,1..3} (4 alike) : Constant  Value=7.5
  Mux : Mux
  Product{,1..23} (24 alike) : Product
  Sum : Sum  Inputs=|++
  Trigonometric Function : Trigonometry
  const {,1..3} (4 alike) : Constant  Value=-1
  x1-a1b1 : Sum  Inputs=+-
  x2-a1b1 : Product
  y2+a1alph1 : Product
  y2+a1alph2 : Product
  y2-a2alph2 : Product
  Ток : Outport
  wires:
  Mux/1 -> Ток/1
  Вектор координат/1 -> Demux/1
  "const "/1 -> Product/2
  Demux/1 -> Add9/1, x1-a1b1/1, Add/1, Add13/1  "x1"
  Product2/1 -> Add/2
  Add/1 -> Product1/2
  Product1/1 -> Add1/1
  Demux/2 -> Add14/1, Add17/1, Add7/1, Add4/2  "y1"
  Demux/3 -> Add11/1, Add2/1  "x2"
  Demux/4 -> Add16/2, Add6/1  "y2"
  Demux/5 -> Product18/2, Product22/2, Product10/2, Product4/1  "alpha1"
  Demux/6 -> Product13/2, Product16/2, Product6/2, Product2/2  "beta1"
  Demux/7 -> Product20/2, Product7/2  "alpha2"
  Demux/8 -> Product14/2, Product3/2  "beta2"
  Product3/1 -> Add2/2
  Add2/1 -> x2-a1b1/1
  x2-a1b1/1 -> Add1/2
  Product6/1 -> x1-a1b1/2
  Add1/1 -> Add3/1
  x1-a1b1/1 -> Integrator/1
  Integrator/1 -> Product5/1
  Product5/1 -> Add3/2
  Add3/1 -> Product/1  "iax"
  Product/1 -> Mux/1  "i_ax"
  Constant/1 -> Product7/1, Product4/2, Product3/1, Product2/1, Product10/1, Product6/1
  Product4/1 -> Add4/1
  Product7/1 -> Add6/2
  Add6/1 -> y2+a1alph2/1
  y2+a1alph2/1 -> Add5/2
  Add4/1 -> Product8/2
  Product8/1 -> Add5/1
  Integrator1/1 -> Product9/1
  Product10/1 -> Add7/2
  Add7/1 -> Integrator1/1
  Product9/1 -> Add8/2
  Add5/1 -> Add8/1
  const 1/1 -> Product11/2
  Add8/1 -> Product11/1
  Product11/1 -> Mux/2  "i_ay"
  Add9/1 -> Product12/2
  Product13/1 -> Add9/2
  Constant1/1 -> Product22/1, Product20/1, Product18/1, Product16/1, Product14/1, Product13/1
  Product12/1 -> Add10/1
  y2+a1alph1/1 -> Add10/2
  Add11/1 -> y2+a1alph1/1
  Product14/1 -> Add11/2
  Add10/1 -> Add12/1
  Integrator2/1 -> Product15/1
  Product15/1 -> Add12/2
  Product16/1 -> Add13/2
  Add13/1 -> Integrator2/1
  const 2/1 -> Product17/2
  Add12/1 -> Product17/1
  Product17/1 -> Mux/3  "i_bx"
  Product18/1 -> Add14/2
  Add14/1 -> Product19/2
  Product19/1 -> Add15/1
  y2-a2alph2/1 -> Add15/2
  Product20/1 -> Add16/1
  Add16/1 -> y2-a2alph2/1
  Add17/1 -> Integrator3/1
  Integrator3/1 -> Product21/1
  Product22/1 -> Add17/2
  const 3/1 -> Product23/2
  Product21/1 -> Product23/1
  Product23/1 -> Mux/4  "i_by"
  Kp/1 -> Product8/1, Product12/1, Product19/1, Product1/1
  Ki/1 -> Product21/2, Product9/2, Product5/2, Product15/2
  "KD "/1 -> x2-a1b1/2, y2+a1alph1/2, y2+a1alph2/2, y2-a2alph2/2

== system Test3/Модель  ==
  In1 : Inport
  Out1 : Outport
  wires:
  In1/1 -> Out1/1

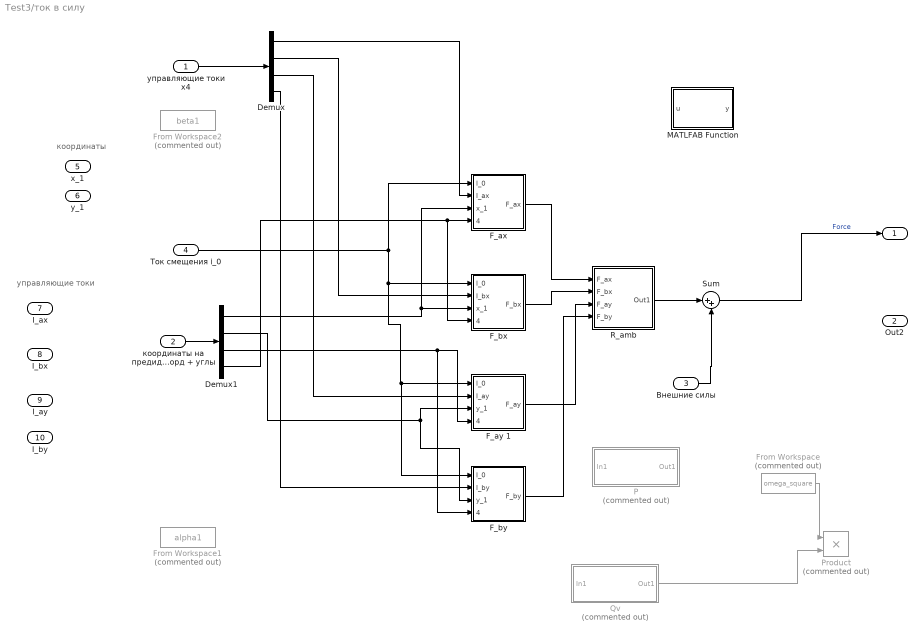
== system Test3/ток в силу  ==
  note: координаты
  note: управляющие токи
  управляющие токи x4 : Inport
  координаты на предидущий такт коорд + углы : Inport  Port=2
  Внешние силы : Inport  Port=3
  Ток смещения i_0 : Inport  Port=4
  x_1 : Inport  Port=5
  y_1 : Inport  Port=6
  I_ax : Inport  Port=7
  I_bx : Inport  Port=8
  I_ay : Inport  Port=9
  I_by : Inport  Port=10
  Demux : Demux
  Demux1 : Demux
  F_ax : Subsystem
  F_ay 1 : Subsystem
  F_bx : Subsystem
  F_by : Subsystem
  From Workspace : FromWorkspace  Commented=on  VariableName=omega_square  SampleTime=0
  From Workspace1 : FromWorkspace  Commented=on  VariableName=alpha1  SampleTime=0
  From Workspace2 : FromWorkspace  Commented=on  VariableName=beta1  SampleTime=0
  MATLFAB Function : MATLAB Function  TreatAsAtomicUnit=on
  P : Subsystem  Commented=on
  Product : Product  Commented=on
  Qv : Subsystem  Commented=on
  R_amb : Subsystem
  Sum : Sum  Inputs=|++
  " " : Outport
  Out2 : Outport  Port=2
  wires:
  F_ax/1(F_ax) -> R_amb/1(F_ax)
  F_bx/1(F_bx) -> R_amb/2(F_bx)
  F_ay 1/1(F_ay) -> R_amb/3(F_ay)
  F_by/1(F_by) -> R_amb/4(F_by)
  R_amb/1(Out1) -> Sum/1
  Sum/1 -> " "/1  "Force"
  From Workspace/1 -> Product/1
  Qv/1(Out1) -> Product/2
  Внешние силы/1 -> Sum/2
  Ток смещения i_0/1 -> F_by/1(I_0), F_ay 1/1(I_0), F_bx/1(I_0), F_ax/1(I_0)
  управляющие токи x4/1 -> Demux/1
  Demux/1 -> F_ax/2(I_ax)
  Demux/2 -> F_bx/2(I_bx)
  Demux/3 -> F_ay 1/2(I_ay)
  Demux/4 -> F_by/2(I_by)
  координаты на предидущий такт коорд + углы/1 -> Demux1/1
  Demux1/1 -> F_ax/3(x_1), F_bx/3(x_1)
  Demux1/2 -> F_by/3(y_1), F_ay 1/3(y_1)
  Demux1/3 -> F_by/4(alpha_1), F_ay 1/4(alpha_1)
  Demux1/4 -> F_bx/4(betta_1), F_ax/4(betta_1)

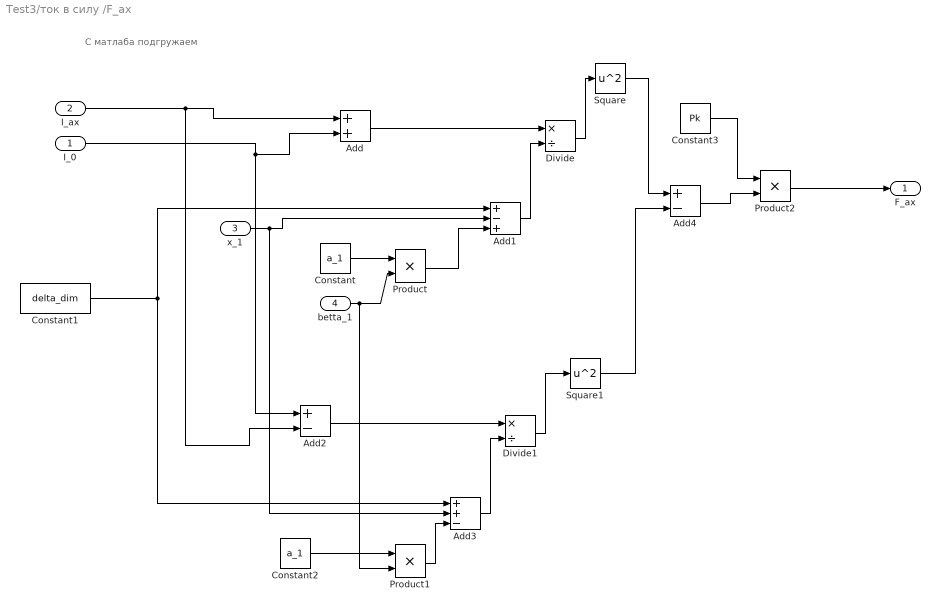
== system Test3/ток в силу /F_ax ==
  note: С матлаба подгружаем
  I_0 : Inport
  I_ax : Inport  Port=2
  x_1 : Inport  Port=3
  betta_1 : Inport  Port=4
  Add : Sum
  Add1 : Sum  Inputs=+-+
  Add2 : Sum  Inputs=+-
  Add3 : Sum  Inputs=++-
  Add4 : Sum  Inputs=+-
  Constant : Constant  Value=a_1
  Constant1 : Constant  Value=delta_dim
  Constant2 : Constant  Value=a_1
  Constant3 : Constant  Value=Pk
  Divide : Product  Inputs=*/
  Divide1 : Product  Inputs=*/
  Product : Product
  Product1 : Product
  Product2 : Product
  Square : Math  Operator=square  SaturateOnIntegerOverflow=on
  Square1 : Math  Operator=square  SaturateOnIntegerOverflow=on
  F_ax : Outport
  wires:
  Product2/1 -> F_ax/1
  Constant/1 -> Product/1
  Product/1 -> Add1/3
  Add1/1 -> Divide/2
  Add/1 -> Divide/1
  Divide/1 -> Square/1
  Product1/1 -> Add3/3
  Add2/1 -> Divide1/1
  Constant2/1 -> Product1/1
  I_ax/1 -> Add2/2, Add/1
  Add3/1 -> Divide1/2
  x_1/1 -> Add1/2, Add3/2
  Divide1/1 -> Square1/1
  I_0/1 -> Add/2, Add2/1
  betta_1/1 -> Product/2, Product1/2
  Square/1 -> Add4/1
  Square1/1 -> Add4/2
  Constant3/1 -> Product2/1
  Add4/1 -> Product2/2
  Constant1/1 -> Add1/1, Add3/1

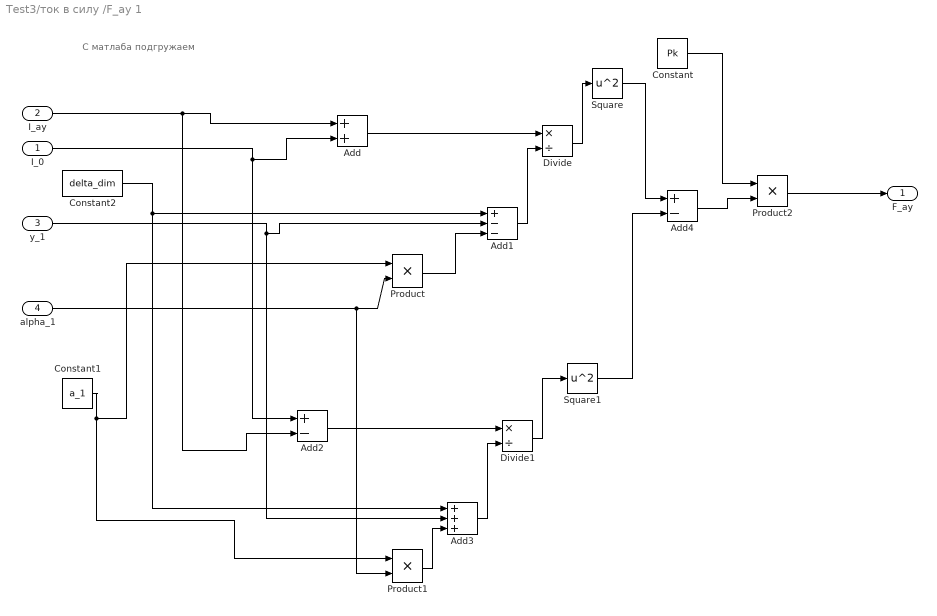
== system Test3/ток в силу /F_ay 1 ==
  note: С матлаба подгружаем
  I_0 : Inport
  I_ay : Inport  Port=2
  y_1 : Inport  Port=3
  alpha_1 : Inport  Port=4
  Add : Sum
  Add1 : Sum  Inputs=+--
  Add2 : Sum  Inputs=+-
  Add3 : Sum  Inputs=+++
  Add4 : Sum  Inputs=+-
  Constant : Constant  Value=Pk
  Constant1 : Constant  Value=a_1
  Constant2 : Constant  Value=delta_dim
  Divide : Product  Inputs=*/
  Divide1 : Product  Inputs=*/
  Product : Product
  Product1 : Product
  Product2 : Product
  Square : Math  Operator=square  SaturateOnIntegerOverflow=on
  Square1 : Math  Operator=square  SaturateOnIntegerOverflow=on
  F_ay : Outport
  wires:
  Product2/1 -> F_ay/1
  Product/1 -> Add1/3
  Add1/1 -> Divide/2
  Add/1 -> Divide/1
  Divide/1 -> Square/1
  Product1/1 -> Add3/3
  Add2/1 -> Divide1/1
  Constant1/1 -> Product1/1, Product/1
  I_ay/1 -> Add2/2, Add/1
  Add3/1 -> Divide1/2
  y_1/1 -> Add1/2, Add3/2
  Divide1/1 -> Square1/1
  I_0/1 -> Add/2, Add2/1
  alpha_1/1 -> Product/2, Product1/2
  Square/1 -> Add4/1
  Square1/1 -> Add4/2
  Constant/1 -> Product2/1
  Add4/1 -> Product2/2
  Constant2/1 -> Add3/1, Add1/1

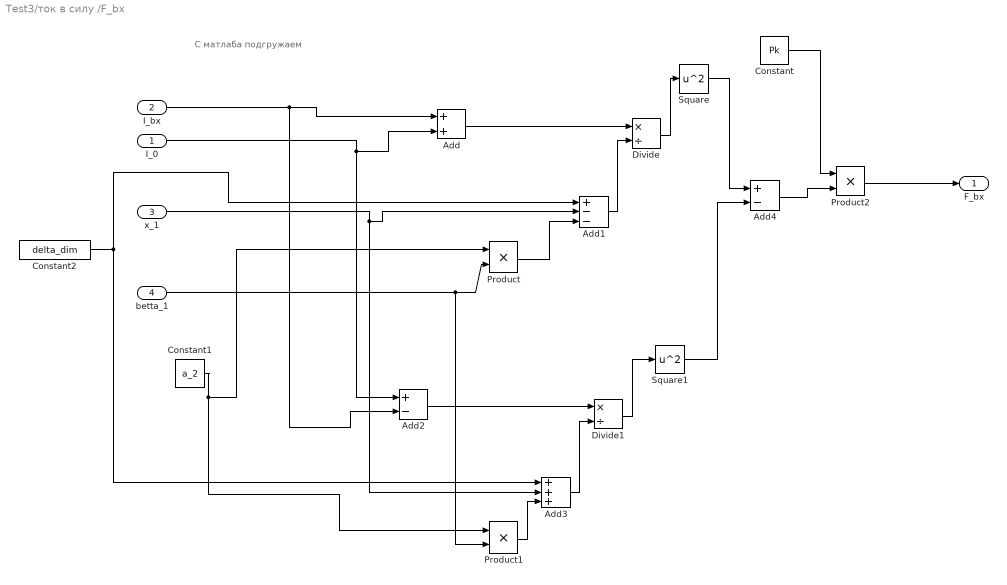
== system Test3/ток в силу /F_bx ==
  note: С матлаба подгружаем
  I_0 : Inport
  I_bx : Inport  Port=2
  x_1 : Inport  Port=3
  betta_1 : Inport  Port=4
  Add : Sum
  Add1 : Sum  Inputs=+--
  Add2 : Sum  Inputs=+-
  Add3 : Sum  Inputs=+++
  Add4 : Sum  Inputs=+-
  Constant : Constant  Value=Pk
  Constant1 : Constant  Value=a_2
  Constant2 : Constant  Value=delta_dim
  Divide : Product  Inputs=*/
  Divide1 : Product  Inputs=*/
  Product : Product
  Product1 : Product
  Product2 : Product
  Square : Math  Operator=square  SaturateOnIntegerOverflow=on
  Square1 : Math  Operator=square  SaturateOnIntegerOverflow=on
  F_bx : Outport
  wires:
  Product2/1 -> F_bx/1
  Product/1 -> Add1/3
  Add1/1 -> Divide/2
  Add/1 -> Divide/1
  Divide/1 -> Square/1
  Product1/1 -> Add3/3
  Add2/1 -> Divide1/1
  Constant1/1 -> Product1/1, Product/1
  I_bx/1 -> Add2/2, Add/1
  Add3/1 -> Divide1/2
  x_1/1 -> Add1/2, Add3/2
  Divide1/1 -> Square1/1
  I_0/1 -> Add/2, Add2/1
  betta_1/1 -> Product/2, Product1/2
  Square/1 -> Add4/1
  Square1/1 -> Add4/2
  Constant/1 -> Product2/1
  Add4/1 -> Product2/2
  Constant2/1 -> Add1/1, Add3/1

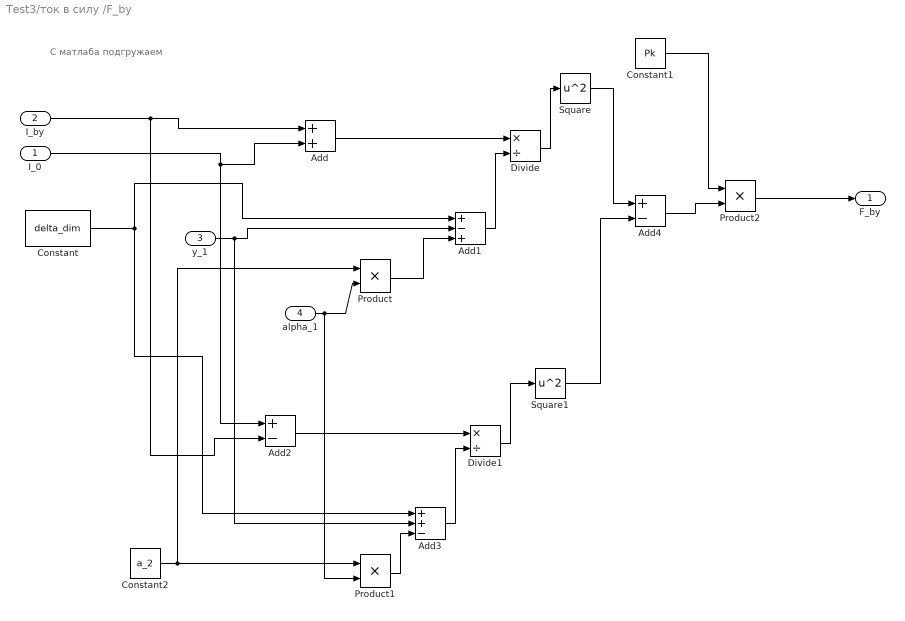
== system Test3/ток в силу /F_by ==
  note: С матлаба подгружаем
  I_0 : Inport
  I_by : Inport  Port=2
  y_1 : Inport  Port=3
  alpha_1 : Inport  Port=4
  Add : Sum
  Add1 : Sum  Inputs=+-+
  Add2 : Sum  Inputs=+-
  Add3 : Sum  Inputs=++-
  Add4 : Sum  Inputs=+-
  Constant : Constant  Value=delta_dim
  Constant1 : Constant  Value=Pk
  Constant2 : Constant  Value=a_2
  Divide : Product  Inputs=*/
  Divide1 : Product  Inputs=*/
  Product : Product
  Product1 : Product
  Product2 : Product
  Square : Math  Operator=square  SaturateOnIntegerOverflow=on
  Square1 : Math  Operator=square  SaturateOnIntegerOverflow=on
  F_by : Outport
  wires:
  Product2/1 -> F_by/1
  Constant2/1 -> Product/1, Product1/1
  Product/1 -> Add1/3
  Add1/1 -> Divide/2
  Add/1 -> Divide/1
  Divide/1 -> Square/1
  Product1/1 -> Add3/3
  Add2/1 -> Divide1/1
  I_by/1 -> Add2/2, Add/1
  Add3/1 -> Divide1/2
  y_1/1 -> Add1/2, Add3/2
  Constant/1 -> Add1/1, Add3/1
  Divide1/1 -> Square1/1
  I_0/1 -> Add/2, Add2/1
  alpha_1/1 -> Product/2, Product1/2
  Square/1 -> Add4/1
  Square1/1 -> Add4/2
  Constant1/1 -> Product2/1
  Add4/1 -> Product2/2

== system Test3/ток в силу /P ==
  In1 : Inport
  Out1 : Outport
  wires:
  In1/1 -> Out1/1

== system Test3/ток в силу /Qv ==
  In1 : Inport
  Out1 : Outport
  wires:
  In1/1 -> Out1/1

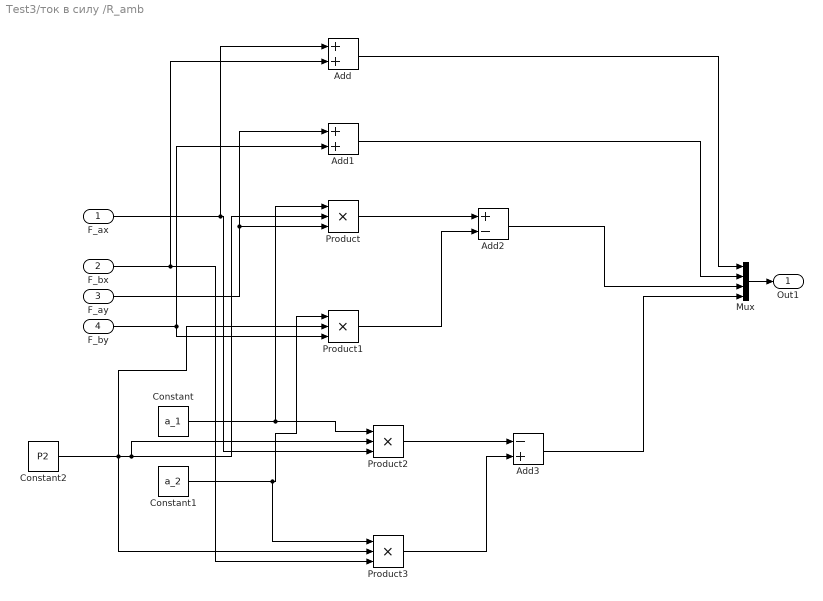
== system Test3/ток в силу /R_amb ==
  F_ax : Inport
  F_bx : Inport  Port=2
  F_ay : Inport  Port=3
  F_by : Inport  Port=4
  Add : Sum
  Add1 : Sum
  Add2 : Sum  Inputs=+-
  Add3 : Sum  Inputs=-+
  Constant : Constant  Value=a_1
  Constant1 : Constant  Value=a_2
  Constant2 : Constant  Value=P2
  Mux : Mux
  Product{,1..3} (4 alike) : Product  Inputs=3
  Out1 : Outport
  wires:
  F_ax/1 -> Product2/3, Add/1
  F_bx/1 -> Product3/3, Add/2
  Add/1 -> Mux/1
  F_ay/1 -> Product/3, Add1/1
  F_by/1 -> Product1/3, Add1/2
  Add1/1 -> Mux/2
  Mux/1 -> Out1/1
  Constant/1 -> Product2/1, Product/1
  Product/1 -> Add2/1
  Constant1/1 -> Product3/1, Product1/1
  Product1/1 -> Add2/2
  Add2/1 -> Mux/3
  Product3/1 -> Add3/2
  Product2/1 -> Add3/1
  Add3/1 -> Mux/4
  Constant2/1 -> Product/2, Product2/2, Product3/2, Product1/2

== matlab function Test3/ток в силу /MATLFAB Function ==
  data: u input; y output
function y = fcn(u)

y = u;
